simulink model "modelPID"  (R2013a)
settings: Solver=ode4  StartTime=0.0  StopTime=time  FixedStep=0.001  MaxStep=2  MinStep=0.01  RelTol=1e-3
values from neighbouring files (symbols this model uses):
  D = I/4    (= 0)    [main.m]
  I = 2/w_osc*tan(1/2*(fi-pi()/4))    [main.m]
  P = 2/Mr*w_osc*I/((w_osc*I)^2 + 4)    [main.m]
  y_zad = 1    [main.m]
libraries: cstblocks x2, simulink x1
settings Model: Creator=Michał Strada  LastModifiedBy=Michał Strada

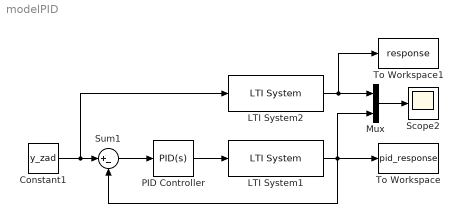
== system modelPID ==
  Constant1 : Constant  Value=y_zad
  LTI System1 : cstblocks/LTI System  sys=G  IC=[]
  LTI System2 : cstblocks/LTI System  sys=G  IC=[]
  Mux : Mux  Inputs=2
  PID Controller : simulink/Continuous/PID Controller  Controller=PID  TimeDomain=Continuous-time  SampleTime=1  IntegratorMethod=Forward Euler  FilterMethod=Forward Euler  Form=Parallel  P=P  I=I  D=D  N=100  InitialConditionSource=internal  InitialConditionForIntegrator=0  InitialConditionForFilter=0  ExternalReset=none  LimitOutput=off  UpperSaturationLimit=inf  LowerSaturationLimit=-inf  LinearizeAsGain=on  AntiWindupMode=none  Kb=1  TrackingMode=off  Kt=1  PParamMin=[]  PParamMax=[]  IParamMin=[]  IParamMax=[]  DParamMin=[]  DParamMax=[]  NParamMin=[]  NParamMax=[]  KbParamMin=[]  KbParamMax=[]  KtParamMin=[]  KtParamMax=[]  POutMin=[]  POutMax=[]  IOutMin=[]  IOutMax=[]  DOutMin=[]  DOutMax=[]  NOutMin=[]  NOutMax=[]  KbOutMin=[]  KbOutMax=[]  KtOutMin=[]  KtOutMax=[]  IntegratorOutMin=[]  IntegratorOutMax=[]  FilterOutMin=[]  FilterOutMax=[]  SumOutMin=[]  SumOutMax=[]  SumI1OutMin=[]  SumI1OutMax=[]  SumI2OutMin=[]  SumI2OutMax=[]  SumI3OutMin=[]  SumI3OutMax=[]  SumDOutMin=[]  SumDOutMax=[]  SaturationOutMin=[]  SaturationOutMax=[]  IntegratorContinuousStateAttributes=''  IntegratorStateMustResolveToSignalObject=off  IntegratorRTWStateStorageClass=Auto  FilterContinuousStateAttributes=''  FilterStateMustResolveToSignalObject=off  FilterRTWStateStorageClass=Auto
  Scope2 : Scope
      settings: MaxDataPoints=500000
  Sum1 : Sum  Inputs=|+-
  To Workspace : ToWorkspace  VariableName=pid_response  SampleTime=-1  SaveFormat=Timeseries
  To Workspace1 : ToWorkspace  VariableName=response  SampleTime=-1  SaveFormat=Timeseries
  wires:
  Mux/1 -> Scope2/1
  LTI System1/1 -> To Workspace/1, Sum1/2, Mux/2
  PID Controller/1 -> LTI System1/1
  LTI System2/1 -> To Workspace1/1, Mux/1
  Constant1/1 -> LTI System2/1, Sum1/1
  Sum1/1 -> PID Controller/1
